simulink model "Seventh_Order_Polynomial_Clean_Test_Harness"  (R2021b)
settings: Solver=FixedStepDiscrete  StartTime=0.0  StopTime=56  FixedStep=0.001  RelTol=1e-3
model workspace (MAT data in the model file):
  mwTaskManagerKernelLatency = 0
libraries: simulink_extras x2
settings Model: Creator=salva  LastModifiedBy=salva
settings DataIOCC: ReturnWorkspaceOutputsName=septic_out
settings OptimizationCC: DefaultParameterBehavior=Inlined  DefaultUnderspecifiedDataType=single  EnhancedBackFolding=on  PassReuseOutputArgsAs=Individual arguments  ZeroExternalMemoryAtStartup=off  ZeroInternalMemoryAtStartup=off  MaxStackSize=64  OptimizeBlockOrder=speed  DifferentSizesBufferReuse=on  OptimizationCustomize=off  EfficientTunableParamExpr=on
settings DebuggingCC: ParameterTunabilityLossMsg=error
settings HardwareCC: ProdBitPerChar=16  ProdBitPerInt=16  ProdBitPerPointer=32  ProdBitPerSizeT=32  ProdBitPerPtrDiffT=32  ProdLargestAtomicInteger=Integer  ProdLargestAtomicFloat=None  ProdWordSize=16  ProdHWDeviceType=Texas Instruments->C2000  HardwareBoardFeatureSet=SoCBlockset
settings ModelReferenceCC: ModelReferenceNumInstancesAllowed=Single
settings SFSimCC: MATLABDynamicMemAlloc=off
settings RTWCC: Description=Embedded Coder  SystemTargetFile=ert.tlc  TemplateMakefile=ert_default_tmf
settings CodeAppCC: ForceParamTrailComments=on  IgnoreCustomStorageClasses=off  OperatorAnnotations=on  SimulinkDataObjDesc=on  SFDataObjDesc=on  InsertBlockDesc=on
settings ERTTargetCC: TargetLangStandard=C99 (ISO)  InlinedParameterPlacement=NonHierarchical  ERTCustomFileTemplate=example_file_process.tlc

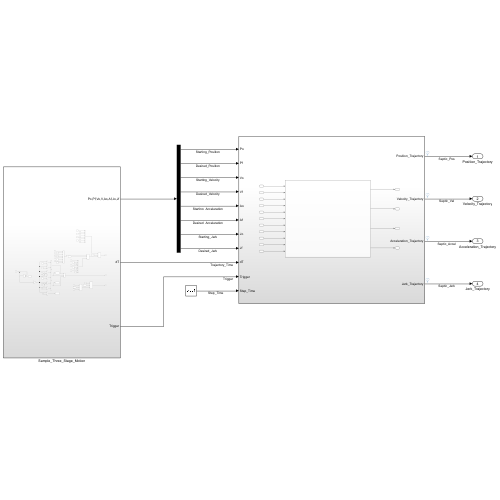
[thumbnail: Simulink's stored preview of the top-level diagram]
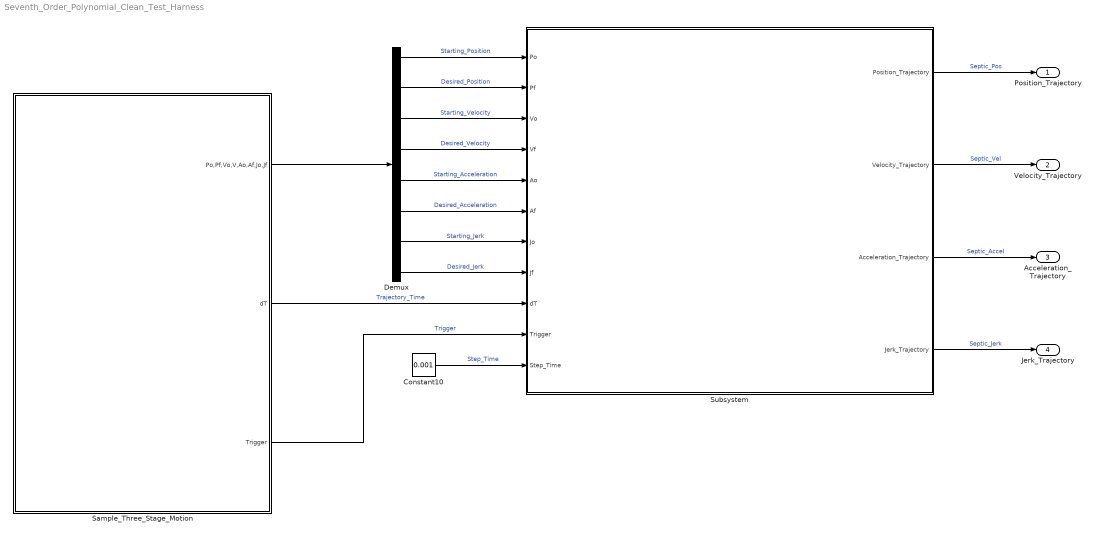
== system Seventh_Order_Polynomial_Clean_Test_Harness ==
  Constant10 : Constant  Value=0.001
  Demux : Demux  Outputs=8
  Sample_Three_Stage_Motion : Subsystem
  Subsystem : Subsystem
  Position_Trajectory : Outport
  Velocity_Trajectory : Outport  Port=2
  Acceleration_Trajectory : Outport  Port=3
  Jerk_Trajectory : Outport  Port=4
  wires:
  Demux/1 -> Subsystem/1(Po)  "Starting_Position"
  Demux/2 -> Subsystem/2(Pf)  "Desired_Position"
  Demux/3 -> Subsystem/3(Vo)  "Starting_Velocity"
  Demux/4 -> Subsystem/4(Vf)  "Desired_Velocity"
  Demux/5 -> Subsystem/5(Ao)  "Starting_Acceleration"
  Demux/6 -> Subsystem/6(Af)  "Desired_Acceleration"
  Demux/7 -> Subsystem/7(Jo)  "Starting_Jerk"
  Demux/8 -> Subsystem/8(Jf)  "Desired_Jerk"
  Constant10/1 -> Subsystem/11(Step_Time)  "Step_Time"
  Subsystem/1(Position_Trajectory) -> Position_Trajectory/1  "Septic_Pos"
  Subsystem/2(Velocity_Trajectory) -> Velocity_Trajectory/1  "Septic_Vel"
  Subsystem/3(Acceleration_Trajectory) -> Acceleration_Trajectory/1  "Septic_Accel"
  Subsystem/4(Jerk_Trajectory) -> Jerk_Trajectory/1  "Septic_Jerk"
  Sample_Three_Stage_Motion/3(Trigger) -> Subsystem/10(Trigger)  "Trigger"
  Sample_Three_Stage_Motion/2(dT) -> Subsystem/9(dT)  "Trajectory_Time"
  Sample_Three_Stage_Motion/1(Po,Pf,Vo,V,Ao,Af,Jo,Jf) -> Demux/1

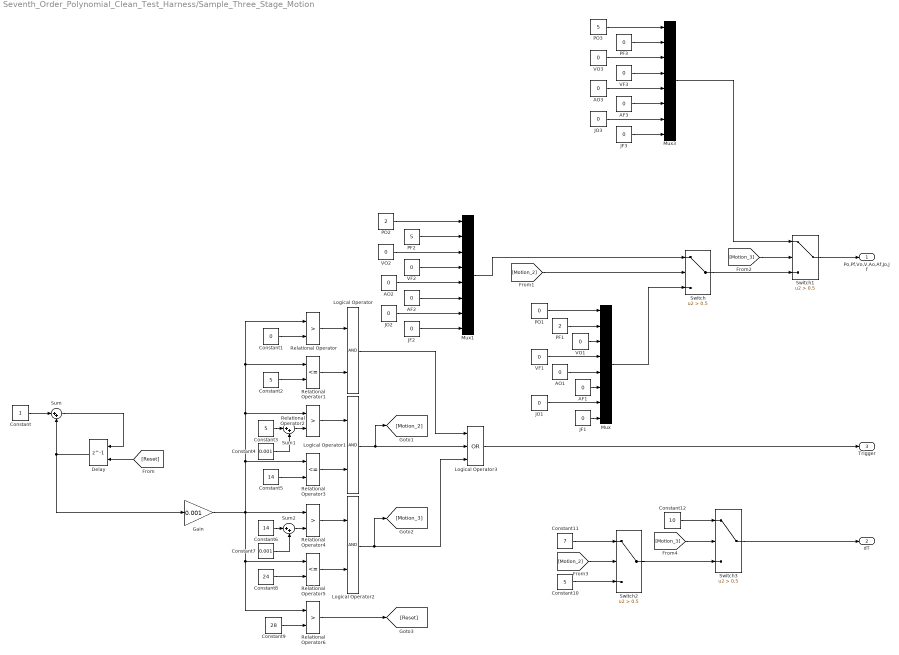
== system Seventh_Order_Polynomial_Clean_Test_Harness/Sample_Three_Stage_Motion ==
  AF1 : Constant  Value=0
  AF2 : Constant  Value=0
  AF3 : Constant  Value=0
  AO1 : Constant  Value=0
  AO2 : Constant  Value=0
  AO3 : Constant  Value=0
  Constant : Constant
  Constant1 : Constant  Value=0
  Constant10 : Constant  Value=5
  Constant11 : Constant  Value=7
  Constant12 : Constant  Value=10
  Constant2 : Constant  Value=5
  Constant3 : Constant  Value=5
  Constant4 : Constant  Value=0.001
  Constant5 : Constant  Value=14
  Constant6 : Constant  Value=14
  Constant7 : Constant  Value=0.001
  Constant8 : Constant  Value=24
  Constant9 : Constant  Value=28
  Delay : Delay  DelayLength=1  ExternalReset=Rising
      settings: InputPortMap=u0,r5
  Gain : Gain  Gain=0.001
  JF1 : Constant  Value=0
  JF2 : Constant  Value=0
  JF3 : Constant  Value=0
  JO1 : Constant  Value=0
  JO2 : Constant  Value=0
  JO3 : Constant  Value=0
  Logical Operator : Logic  AllPortsSameDT=off  OutDataTypeStr=boolean
  Logical Operator1 : Logic  AllPortsSameDT=off  OutDataTypeStr=boolean
  Logical Operator2 : Logic  AllPortsSameDT=off  OutDataTypeStr=boolean
  Logical Operator3 : Logic  Operator=OR  Inputs=3  AllPortsSameDT=off  OutDataTypeStr=boolean
  Mux : Mux  Inputs=8
  Mux1 : Mux  Inputs=8
  Mux3 : Mux  Inputs=8
  PF1 : Constant  Value=2
  PF2 : Constant  Value=5
  PF3 : Constant  Value=0
  PO1 : Constant  Value=0
  PO2 : Constant  Value=2
  PO3 : Constant  Value=5
  Relational Operator{,2,4,6} (4 alike) : RelationalOperator  Operator=>  OutDataTypeStr=boolean  RndMeth=Simplest
  Relational Operator1 : RelationalOperator  Operator=<=  OutDataTypeStr=boolean  RndMeth=Simplest
  Relational Operator3 : RelationalOperator  Operator=<=  OutDataTypeStr=boolean  RndMeth=Simplest
  Relational Operator5 : RelationalOperator  Operator=<=  OutDataTypeStr=boolean  RndMeth=Simplest
  Sum : Sum  Inputs=|++
  Sum1 : Sum  Inputs=|++
  Sum2 : Sum  Inputs=|++
  Switch{,1..3} (4 alike) : Switch  Criteria=u2 > Threshold  Threshold=0.5
  VF1 : Constant  Value=0
  VF2 : Constant  Value=0
  VF3 : Constant  Value=0
  VO1 : Constant  Value=0
  VO2 : Constant  Value=0
  VO3 : Constant  Value=0
  Po,Pf,Vo,V,Ao,Af,Jo,Jf : Outport
  dT : Outport  Port=2
  Trigger : Outport  Port=3
  wires:
  VF2/1 -> Mux1/4
  Delay/1 -> Sum/2, Gain/1
  Sum1/1 -> Relational Operator2/2
  Constant3/1 -> Sum1/1
  Constant1/1 -> Relational Operator/2
  VO2/1 -> Mux1/3
  Gain/1 -> Relational Operator/1, Relational Operator1/1, Relational Operator2/1, Relational Operator3/1, Relational Operator6/1, Relational Operator5/1, Relational Operator4/1
  Switch1/1 -> Po,Pf,Vo,V,Ao,Af,Jo,Jf/1
  Relational Operator3/1 -> Logical Operator1/2
  Switch/1 -> Switch1/3
  Constant/1 -> Sum/1
  Logical Operator2/1 -> [Motion_3], Logical Operator3/3
  Sum2/1 -> Relational Operator4/2
  PO1/1 -> Mux/1
  [Motion_2] -> Switch/2
  VF1/1 -> Mux/4
  Constant6/1 -> Sum2/1
  Constant8/1 -> Relational Operator5/2
  Constant7/1 -> Sum2/2
  Constant9/1 -> Relational Operator6/2
  Relational Operator1/1 -> Logical Operator/2
  PO3/1 -> Mux3/1
  Relational Operator/1 -> Logical Operator/1
  Relational Operator5/1 -> Logical Operator2/2
  [Reset] -> Delay/2
  Mux3/1 -> Switch1/1
  Relational Operator4/1 -> Logical Operator2/1
  Sum/1 -> Delay/1
  Mux1/1 -> Switch/1
  PF3/1 -> Mux3/2
  Constant4/1 -> Sum1/2
  VF3/1 -> Mux3/4
  Logical Operator1/1 -> [Motion_2], Logical Operator3/2
  [Motion_3] -> Switch1/2
  Constant2/1 -> Relational Operator1/2
  VO3/1 -> Mux3/3
  Logical Operator3/1 -> Trigger/1
  Logical Operator/1 -> Logical Operator3/1
  Constant5/1 -> Relational Operator3/2
  Mux/1 -> Switch/3
  PF2/1 -> Mux1/2
  PO2/1 -> Mux1/1
  Relational Operator2/1 -> Logical Operator1/1
  Relational Operator6/1 -> [Reset]
  PF1/1 -> Mux/2
  VO1/1 -> Mux/3
  [Motion_2] -> Switch2/2
  Switch2/1 -> Switch3/3
  [Motion_3] -> Switch3/2
  Constant10/1 -> Switch2/3
  Constant11/1 -> Switch2/1
  Constant12/1 -> Switch3/1
  Switch3/1 -> dT/1
  AO1/1 -> Mux/5
  AF1/1 -> Mux/6
  JO1/1 -> Mux/7
  JF1/1 -> Mux/8
  JO2/1 -> Mux1/7
  JF2/1 -> Mux1/8
  AF2/1 -> Mux1/6
  AO2/1 -> Mux1/5
  JF3/1 -> Mux3/8
  JO3/1 -> Mux3/7
  AO3/1 -> Mux3/5
  AF3/1 -> Mux3/6

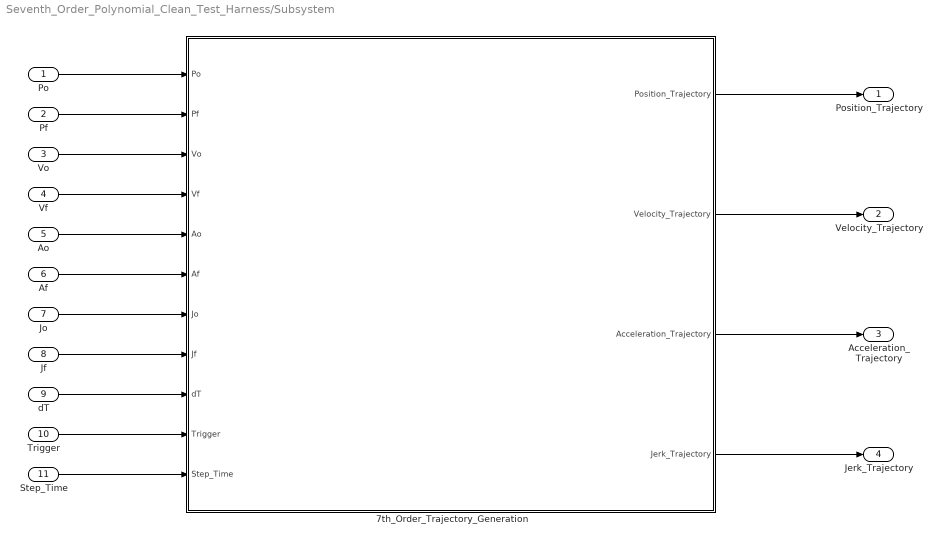
== system Seventh_Order_Polynomial_Clean_Test_Harness/Subsystem ==
  Po : Inport
  Pf : Inport  Port=2
  Vo : Inport  Port=3
  Vf : Inport  Port=4
  Ao : Inport  Port=5
  Af : Inport  Port=6
  Jo : Inport  Port=7
  Jf : Inport  Port=8
  dT : Inport  Port=9
  Trigger : Inport  Port=10
  Step_Time : Inport  Port=11
  7th_Order_Trajectory_Generation : Subsystem
  Position_Trajectory : Outport
  Velocity_Trajectory : Outport  Port=2
  Acceleration_Trajectory : Outport  Port=3
  Jerk_Trajectory : Outport  Port=4
  wires:
  7th_Order_Trajectory_Generation/4(Jerk_Trajectory) -> Jerk_Trajectory/1
  Trigger/1 -> 7th_Order_Trajectory_Generation/10(Trigger)
  Ao/1 -> 7th_Order_Trajectory_Generation/5(Ao)
  Pf/1 -> 7th_Order_Trajectory_Generation/2(Pf)
  Af/1 -> 7th_Order_Trajectory_Generation/6(Af)
  Vo/1 -> 7th_Order_Trajectory_Generation/3(Vo)
  7th_Order_Trajectory_Generation/1(Position_Trajectory) -> Position_Trajectory/1
  dT/1 -> 7th_Order_Trajectory_Generation/9(dT)
  Po/1 -> 7th_Order_Trajectory_Generation/1(Po)
  7th_Order_Trajectory_Generation/2(Velocity_Trajectory) -> Velocity_Trajectory/1
  Vf/1 -> 7th_Order_Trajectory_Generation/4(Vf)
  7th_Order_Trajectory_Generation/3(Acceleration_Trajectory) -> Acceleration_Trajectory/1
  Step_Time/1 -> 7th_Order_Trajectory_Generation/11(Step_Time)
  Jf/1 -> 7th_Order_Trajectory_Generation/8(Jf)
  Jo/1 -> 7th_Order_Trajectory_Generation/7(Jo)

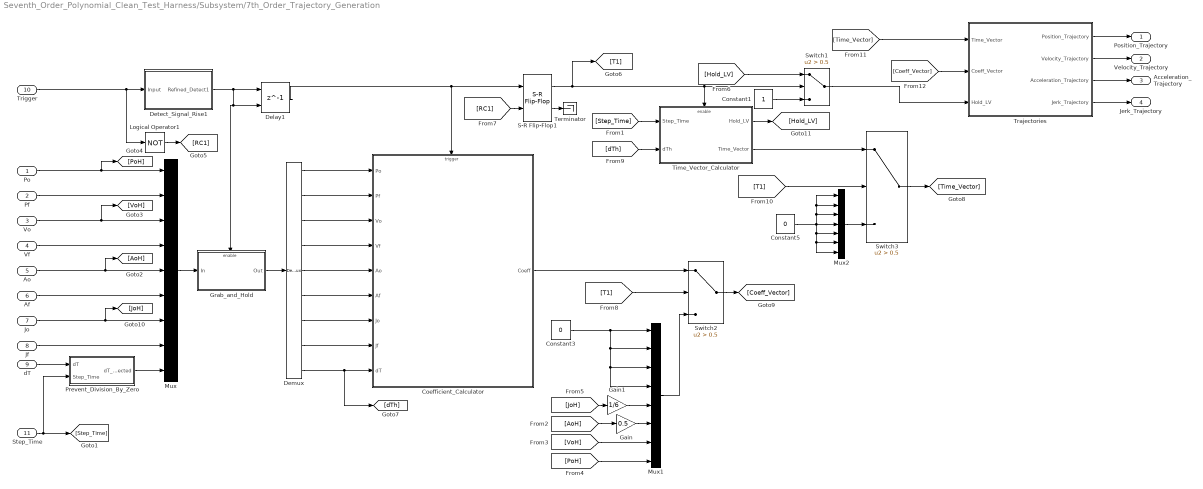
== system Seventh_Order_Polynomial_Clean_Test_Harness/Subsystem/7th_Order_Trajectory_Generation ==
  Po : Inport
  Pf : Inport  Port=2
  Vo : Inport  Port=3
  Vf : Inport  Port=4
  Ao : Inport  Port=5
  Af : Inport  Port=6
  Jo : Inport  Port=7
  Jf : Inport  Port=8
  dT : Inport  Port=9
  Trigger : Inport  Port=10
  Step_Time : Inport  Port=11
  Coefficient_Calculator : Subsystem
  Constant1 : Constant
  Constant3 : Constant  Value=0
  Constant5 : Constant  Value=0
  Delay1 : Delay  DelayLength=1  InitialConditionSource=Input port
      settings: InputPortMap=u0,p4
  Demux : Demux  Outputs=9
  Detect_Signal_Rise1 : Subsystem
  Gain : Gain  Gain=0.5
  Gain1 : Gain  Gain=1/6
  Grab_and_Hold : Subsystem
  Logical Operator1 : Logic  Operator=NOT  AllPortsSameDT=off  OutDataTypeStr=boolean
  Mux : Mux  Inputs=9
  Mux1 : Mux  Inputs=8
  Mux2 : Mux  Inputs=7
  Prevent_Division_By_Zero : Subsystem
  S-R Flip-Flop1 : simulink_extras/Flip Flops/S-R Flip-Flop  initial_condition=0
  Switch1 : Switch  Criteria=u2 > Threshold  Threshold=0.5
  Switch2 : Switch  Criteria=u2 > Threshold  Threshold=0.5
  Switch3 : Switch  Criteria=u2 > Threshold  Threshold=0.5
  Terminator : Terminator
  Time_Vector_Calculator : Subsystem
  Trajectories : Subsystem
  Position_Trajectory : Outport
  Velocity_Trajectory : Outport  Port=2
  Acceleration_Trajectory : Outport  Port=3
  Jerk_Trajectory : Outport  Port=4
  wires:
  Trajectories/2(Velocity_Trajectory) -> Velocity_Trajectory/1
  Trajectories/1(Position_Trajectory) -> Position_Trajectory/1
  [Coeff_Vector] -> Trajectories/2(Coeff_Vector)
  [Time_Vector] -> Trajectories/1(Time_Vector)
  Switch2/1 -> [Coeff_Vector]
  Switch3/1 -> [Time_Vector]
  Constant5/1 -> Mux2/1, Mux2/2, Mux2/3, Mux2/4, Mux2/7, Mux2/6, Mux2/5
  Mux2/1 -> Switch3/3
  Time_Vector_Calculator/2(Time_Vector) -> Switch3/1
  [T1] -> Switch3/2
  [dTh] -> Time_Vector_Calculator/2(dTh)
  [Step_Time] -> Time_Vector_Calculator/1(Step_Time)
  Coefficient_Calculator/1(Coeff) -> Switch2/1
  [T1] -> Switch2/2
  Mux1/1 -> Switch2/3
  S-R Flip-Flop1/1 -> Switch1/2, Time_Vector_Calculator/Enable, [T1]
  S-R Flip-Flop1/2 -> Terminator/1
  [RC1] -> S-R Flip-Flop1/2
  Logical Operator1/1 -> [RC1]
  Delay1/1 -> Coefficient_Calculator/Trigger, S-R Flip-Flop1/1
  Mux/1 -> Grab_and_Hold/1(In)
  Detect_Signal_Rise1/1(Refined_Detect1) -> Delay1/1, Delay1/2, Grab_and_Hold/Enable
  Trigger/1 -> Detect_Signal_Rise1/1(Input), Logical Operator1/1
  Po/1 -> [PoH], Mux/1
  Pf/1 -> Mux/2
  Vo/1 -> [VoH], Mux/3
  Vf/1 -> Mux/4
  Ao/1 -> [AoH], Mux/5
  Af/1 -> Mux/6
  dT/1 -> Prevent_Division_By_Zero/1(dT)
  Grab_and_Hold/1(Out) -> Demux/1
  Trajectories/3(Acceleration_Trajectory) -> Acceleration_Trajectory/1
  Step_Time/1 -> Prevent_Division_By_Zero/2(Step_Time), [Step_Time]
  Prevent_Division_By_Zero/1(dT_Protected) -> Mux/9
  Constant3/1 -> Mux1/4, Mux1/3, Mux1/2, Mux1/1
  [AoH] -> Gain/1
  Jo/1 -> [JoH], Mux/7
  Jf/1 -> Mux/8
  Demux/1 -> Coefficient_Calculator/1(Po)
  Demux/2 -> Coefficient_Calculator/2(Pf)
  Demux/3 -> Coefficient_Calculator/3(Vo)
  Demux/4 -> Coefficient_Calculator/4(Vf)
  Demux/5 -> Coefficient_Calculator/5(Ao)
  Demux/6 -> Coefficient_Calculator/6(Af)
  Demux/7 -> Coefficient_Calculator/7(Jo)
  Demux/8 -> Coefficient_Calculator/8(Jf)
  Demux/9 -> [dTh], Coefficient_Calculator/9(dT)
  [JoH] -> Gain1/1
  Gain1/1 -> Mux1/5
  Gain/1 -> Mux1/6
  [VoH] -> Mux1/7
  [PoH] -> Mux1/8
  Trajectories/4(Jerk_Trajectory) -> Jerk_Trajectory/1
  [Hold_LV] -> Switch1/1
  Switch1/1 -> Trajectories/3(Hold_LV)
  Time_Vector_Calculator/1(Hold_LV) -> [Hold_LV]
  Constant1/1 -> Switch1/3

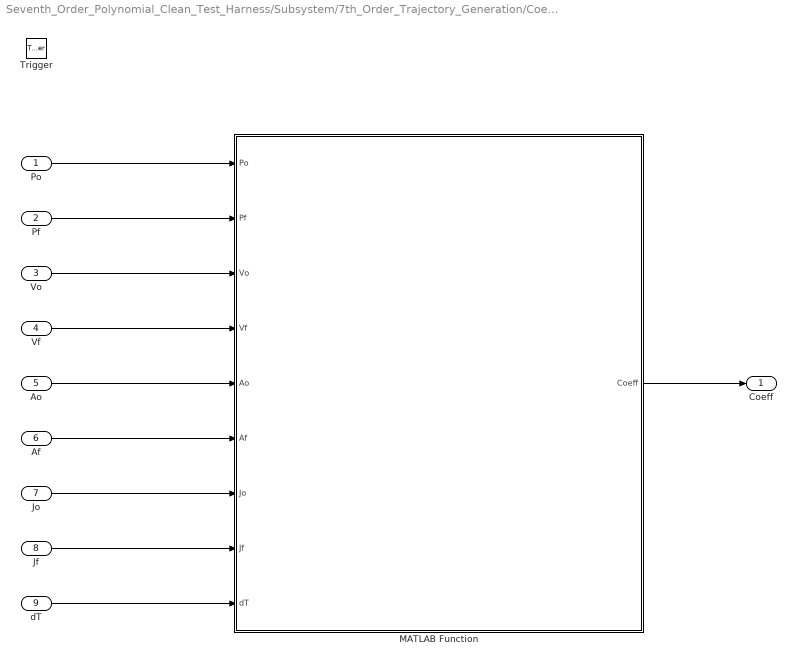
== system Seventh_Order_Polynomial_Clean_Test_Harness/Subsystem/7th_Order_Trajectory_Generation/Coefficient_Calculator ==
  Po : Inport
  Pf : Inport  Port=2
  Vo : Inport  Port=3
  Vf : Inport  Port=4
  Ao : Inport  Port=5
  Af : Inport  Port=6
  Jo : Inport  Port=7
  Jf : Inport  Port=8
  dT : Inport  Port=9
  Trigger : TriggerPort  VariantControl=(inherit)
  MATLAB Function : MATLAB Function  TreatAsAtomicUnit=on
  Coeff : Outport
  wires:
  MATLAB Function/1(Coeff) -> Coeff/1
  Pf/1 -> MATLAB Function/2(Pf)
  Vf/1 -> MATLAB Function/4(Vf)
  Vo/1 -> MATLAB Function/3(Vo)
  Po/1 -> MATLAB Function/1(Po)
  dT/1 -> MATLAB Function/9(dT)
  Ao/1 -> MATLAB Function/5(Ao)
  Af/1 -> MATLAB Function/6(Af)
  Jo/1 -> MATLAB Function/7(Jo)
  Jf/1 -> MATLAB Function/8(Jf)

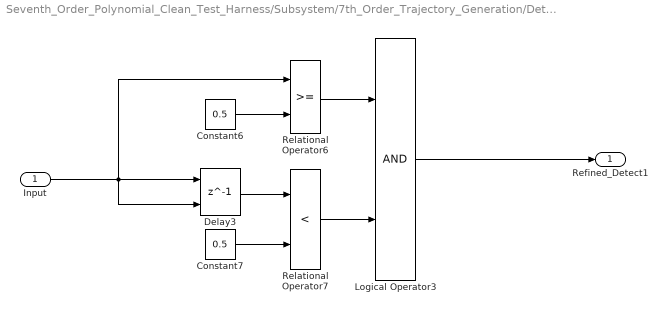
== system Seventh_Order_Polynomial_Clean_Test_Harness/Subsystem/7th_Order_Trajectory_Generation/Detect_Signal_Rise1 ==
  Input : Inport
  Constant6 : Constant  Value=0.5
  Constant7 : Constant  Value=0.5
  Delay3 : Delay  DelayLength=1  InitialConditionSource=Input port
      settings: InputPortMap=u0,p4
  Logical Operator3 : Logic  AllPortsSameDT=off  OutDataTypeStr=boolean
  Relational Operator6 : RelationalOperator  OutDataTypeStr=boolean  RndMeth=Simplest
  Relational Operator7 : RelationalOperator  Operator=<  OutDataTypeStr=boolean  RndMeth=Simplest
  Refined_Detect1 : Outport
  wires:
  Delay3/1 -> Relational Operator7/1
  Relational Operator7/1 -> Logical Operator3/2
  Relational Operator6/1 -> Logical Operator3/1
  Input/1 -> Delay3/2, Delay3/1, Relational Operator6/1
  Constant7/1 -> Relational Operator7/2
  Constant6/1 -> Relational Operator6/2
  Logical Operator3/1 -> Refined_Detect1/1

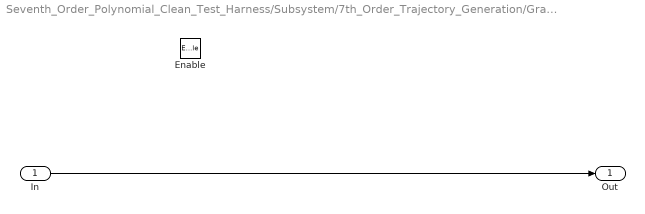
== system Seventh_Order_Polynomial_Clean_Test_Harness/Subsystem/7th_Order_Trajectory_Generation/Grab_and_Hold ==
  In : Inport
  Enable : EnablePort  StatesWhenEnabling=reset
  Out : Outport
  wires:
  In/1 -> Out/1

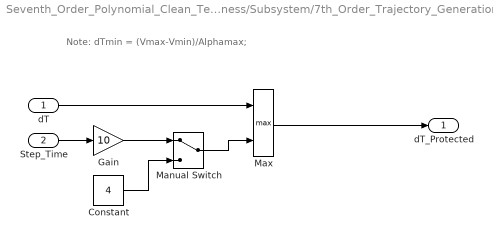
== system Seventh_Order_Polynomial_Clean_Test_Harness/Subsystem/7th_Order_Trajectory_Generation/Prevent_Division_By_Zero ==
  note: Note: dTmin = (Vmax-Vmin)/Alphamax;
  dT : Inport
  Step_Time : Inport  Port=2
  Constant : Constant  Value=4
  Gain : Gain  Gain=10
  Manual Switch : ManualSwitch
  Max : MinMax  Function=max  Inputs=2
  dT_Protected : Outport
  wires:
  dT/1 -> Max/1
  Step_Time/1 -> Gain/1
  Gain/1 -> Manual Switch/1
  Max/1 -> dT_Protected/1
  Manual Switch/1 -> Max/2
  Constant/1 -> Manual Switch/2

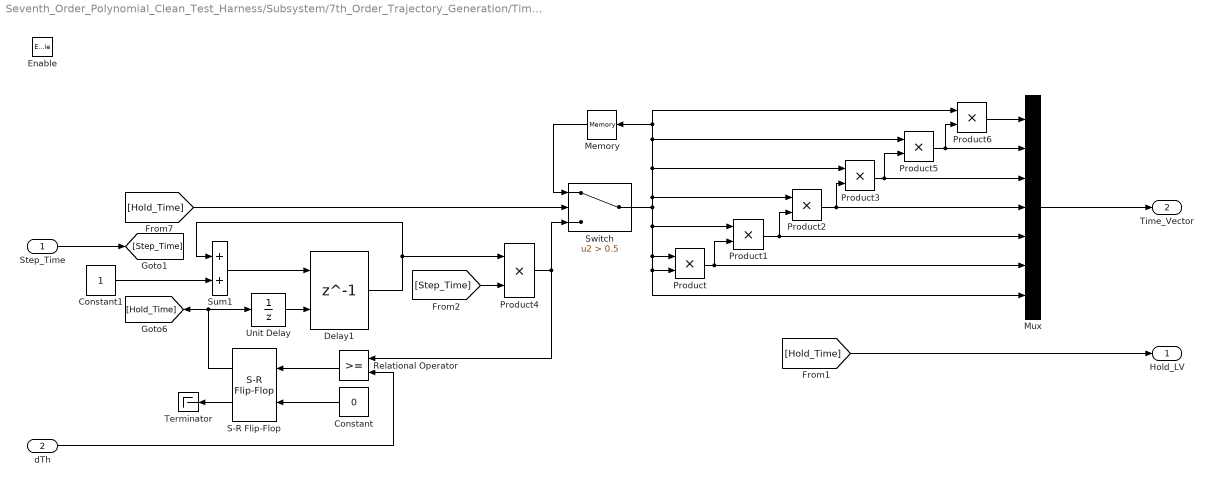
== system Seventh_Order_Polynomial_Clean_Test_Harness/Subsystem/7th_Order_Trajectory_Generation/Time_Vector_Calculator ==
  Step_Time : Inport
  dTh : Inport  Port=2
  Enable : EnablePort  StatesWhenEnabling=reset
  Constant : Constant  Value=0  OutDataTypeStr=boolean
  Constant1 : Constant
  Delay1 : Delay  DelayLength=1  ExternalReset=Level hold
      settings: InputPortMap=u0,r5
  Memory : Memory
  Mux : Mux  Inputs=7
  Product{,1..6} (7 alike) : Product
  Relational Operator : RelationalOperator  OutDataTypeStr=boolean  RndMeth=Simplest
  S-R Flip-Flop : simulink_extras/Flip Flops/S-R Flip-Flop  initial_condition=0
  Sum1 : Sum
  Switch : Switch  Criteria=u2 > Threshold  Threshold=0.5
  Terminator : Terminator
  Unit Delay : UnitDelay  SampleTime=-1  HasFrameUpgradeWarning=on
  Hold_LV : Outport
  Time_Vector : Outport  Port=2
  wires:
  [Hold_Time] -> Hold_LV/1
  Memory/1 -> Switch/1
  Switch/1 -> Product1/1, Product/1, Mux/7, Product/2, Product6/1, Memory/1, Product5/1, Product3/1, Product2/1
  [Hold_Time] -> Switch/2
  Unit Delay/1 -> Delay1/2
  S-R Flip-Flop/1 -> [Hold_Time], Unit Delay/1
  S-R Flip-Flop/2 -> Terminator/1
  Constant/1 -> S-R Flip-Flop/2
  Relational Operator/1 -> S-R Flip-Flop/1
  Mux/1 -> Time_Vector/1
  Product/1 -> Product1/2, Mux/6
  dTh/1 -> Relational Operator/2
  Delay1/1 -> Sum1/1, Product4/1
  Sum1/1 -> Delay1/1
  Product1/1 -> Product2/2, Mux/5
  Product2/1 -> Product3/2, Mux/4
  Step_Time/1 -> [Step_Time]
  Constant1/1 -> Sum1/2
  [Step_Time] -> Product4/2
  Product4/1 -> Switch/3, Relational Operator/1
  Product3/1 -> Product5/2, Mux/3
  Product5/1 -> Product6/2, Mux/2
  Product6/1 -> Mux/1

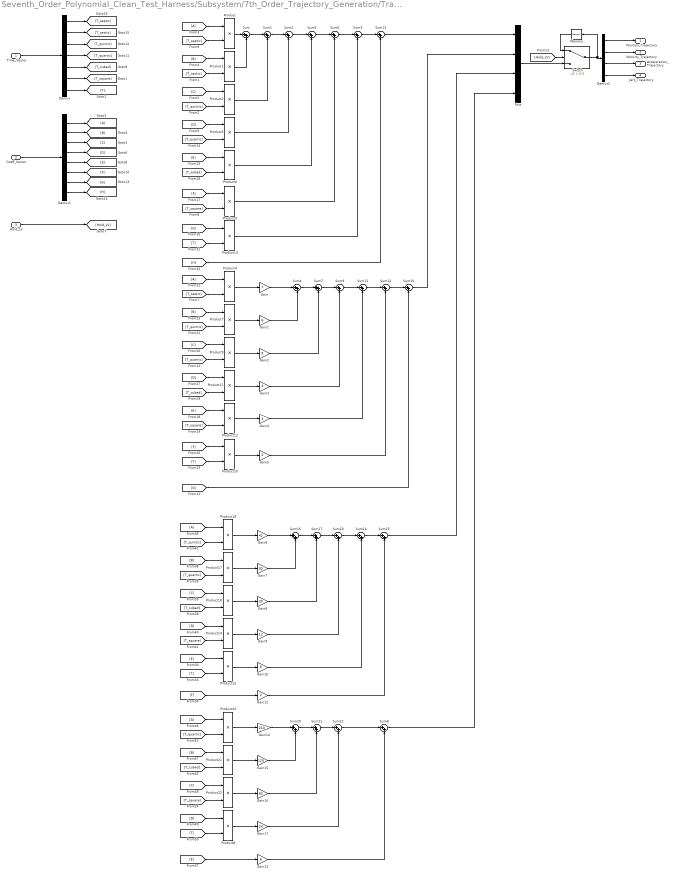
== system Seventh_Order_Polynomial_Clean_Test_Harness/Subsystem/7th_Order_Trajectory_Generation/Trajectories ==
  Time_Vector : Inport
  Coeff_Vector : Inport  Port=2
  Hold_LV : Inport  Port=3
  Demux : Demux  Outputs=7
  Demux1 : Demux  Outputs=8
  Demux2 : Demux
  Gain : Gain  Gain=7
  Gain1 : Gain  Gain=6
  Gain10 : Gain  Gain=6
  Gain11 : Gain  Gain=2
  Gain12 : Gain  Gain=6
  Gain14 : Gain  Gain=210
  Gain15 : Gain  Gain=120
  Gain16 : Gain  Gain=60
  Gain17 : Gain  Gain=24
  Gain2 : Gain  Gain=5
  Gain3 : Gain  Gain=4
  Gain4 : Gain  Gain=3
  Gain5 : Gain  Gain=2
  Gain6 : Gain  Gain=42
  Gain7 : Gain  Gain=30
  Gain8 : Gain  Gain=20
  Gain9 : Gain  Gain=12
  Memory : Memory
  Mux : Mux
  Product{,1..18,20..22} (22 alike) : Product
  Sum{,1..18,20..22} (22 alike) : Sum  Inputs=|++
  Switch : Switch  Criteria=u2 > Threshold  Threshold=0.5
  Position_Trajectory : Outport
  Velocity_Trajectory : Outport  Port=2
  Acceleration_Trajectory : Outport  Port=3
  Jerk_Trajectory : Outport  Port=4
  wires:
  Demux2/2 -> Velocity_Trajectory/1
  Demux2/1 -> Position_Trajectory/1
  [Hold_LV] -> Switch/2
  Memory/1 -> Switch/1
  Switch/1 -> Memory/1, Demux2/1
  Hold_LV/1 -> [Hold_LV]
  Mux/1 -> Switch/3
  Sum1/1 -> Sum2/1
  Product2/1 -> Sum1/2
  [T_quintic] -> Product2/2
  [C] -> Product2/1
  Sum/1 -> Sum1/1
  Product1/1 -> Sum/2
  [T_sextic] -> Product1/2
  [B] -> Product1/1
  Product/1 -> Sum/1
  [T_septic] -> Product/2
  [A] -> Product/1
  Demux1/4 -> [D]
  Demux1/3 -> [C]
  Demux1/2 -> [B]
  Demux1/1 -> [A]
  Coeff_Vector/1 -> Demux1/1
  Time_Vector/1 -> Demux/1
  Demux1/5 -> [E]
  Demux1/6 -> [F]
  [D] -> Product5/1
  [T_quartic] -> Product5/2
  Product5/1 -> Sum2/2
  Sum2/1 -> Sum5/1
  Product6/1 -> Sum5/2
  [E] -> Product6/1
  [T_cubed] -> Product6/2
  Sum5/1 -> Sum6/1
  Demux2/3 -> Acceleration_Trajectory/1
  Demux1/7 -> [G]
  Demux1/8 -> [H]
  Demux/7 -> [T]
  Demux/6 -> [T_square]
  Demux/5 -> [T_cubed]
  Demux/4 -> [T_quartic]
  Demux/3 -> [T_quintic]
  Demux/2 -> [T_sextic]
  Demux/1 -> [T_septic]
  [F] -> Product3/1
  [T_square] -> Product3/2
  Product3/1 -> Sum6/2
  Sum6/1 -> Sum3/1
  [G] -> Product13/1
  [T] -> Product13/2
  Product13/1 -> Sum3/2
  Sum3/1 -> Sum13/1
  [H] -> Sum13/2
  Product10/1 -> Gain5/1
  [T] -> Product10/2
  [F] -> Product10/1
  [G] -> Sum10/2
  Product4/1 -> Gain/1
  [A] -> Product4/1
  Sum4/1 -> Sum7/1
  [E] -> Product12/1
  Product12/1 -> Gain4/1
  Sum11/1 -> Sum12/1
  Sum12/1 -> Sum10/1
  [D] -> Product11/1
  [C] -> Product9/1
  Product11/1 -> Gain3/1
  Sum7/1 -> Sum9/1
  Product9/1 -> Gain2/1
  Product7/1 -> Gain1/1
  Sum9/1 -> Sum11/1
  [B] -> Product7/1
  Gain/1 -> Sum4/1
  [T_sextic] -> Product4/2
  Gain1/1 -> Sum4/2
  [T_quintic] -> Product7/2
  [T_quartic] -> Product9/2
  Gain2/1 -> Sum7/2
  Gain3/1 -> Sum9/2
  [T_cubed] -> Product11/2
  [T_square] -> Product12/2
  Gain4/1 -> Sum11/2
  Gain5/1 -> Sum12/2
  Gain11/1 -> Sum15/2
  Gain10/1 -> Sum14/2
  Sum18/1 -> Sum14/1
  Product14/1 -> Gain9/1
  Product18/1 -> Gain8/1
  [B] -> Product17/1
  Sum17/1 -> Sum18/1
  Sum16/1 -> Sum17/1
  [E] -> Product15/1
  [C] -> Product18/1
  Sum14/1 -> Sum15/1
  Product15/1 -> Gain10/1
  [D] -> Product14/1
  [F] -> Gain11/1
  [T_quintic] -> Product16/2
  [T_cubed] -> Product18/2
  Product17/1 -> Gain7/1
  Gain7/1 -> Sum16/2
  Product16/1 -> Gain6/1
  Gain6/1 -> Sum16/1
  [T_quartic] -> Product17/2
  Gain9/1 -> Sum18/2
  [T_square] -> Product14/2
  Gain8/1 -> Sum17/2
  [T] -> Product15/2
  [A] -> Product16/1
  Sum13/1 -> Mux/1
  Sum10/1 -> Mux/2
  Sum15/1 -> Mux/3
  [A] -> Product20/1
  Gain16/1 -> Sum21/2
  [T] -> Product8/2
  Gain17/1 -> Sum22/2
  [T_cubed] -> Product21/2
  Gain14/1 -> Sum20/1
  Product20/1 -> Gain14/1
  Gain15/1 -> Sum20/2
  Product21/1 -> Gain15/1
  [T_square] -> Product22/2
  [T_quartic] -> Product20/2
  [D] -> Product8/1
  [E] -> Gain12/1
  [C] -> Product22/1
  Sum20/1 -> Sum21/1
  Sum21/1 -> Sum22/1
  [B] -> Product21/1
  Product22/1 -> Gain16/1
  Product8/1 -> Gain17/1
  Sum22/1 -> Sum8/1
  Gain12/1 -> Sum8/2
  Sum8/1 -> Mux/4
  Demux2/4 -> Jerk_Trajectory/1

== matlab function Seventh_Order_Polynomial_Clean_Test_Harness/Subsystem/7th_Order_Trajectory_Generation/Coefficient_Calculator/MATLAB Function ==
  data: Po input; Coeff output; Pf input; Vo input; Vf input; Ao input; Af input; Jo input; Jf input; dT input
function Coeff = solve_septic(Po, Pf, Vo, Vf, Ao, Af, Jo, Jf, dT)

% Position = (A)*dT^7 + (B)*dT^6 + (C)*dT^5 + (D)*dT^4 + (E)*dT^3 + (F)*dT^2 + (G)*dT+ H;
% Velocity = (7*A)*dT^6 + (6*B)*dT^5 + (5*C)*dT^4 + (4*D)*dT^3 + (3*E)*dT^2 + (2*F)*dT+ (G);
% Acceleration = (42*A)*dT^5 + (30*B)*dT^4 + (20*C)*dT^3 + (12*D)*dT^2 + (6*E)*dT + (2*F);
% Jerk = (210*A)*dT^4 + (120*B)*dT^3 + (60*C)*dT^2 + (24*D)*dT + (6*E);
% Where P(t=0) = Po; P(t=dT) = Pf; V(t=0)=Vo; V(t=dT) = Vf; A(t=0) = Ao;
% A(t=dT) = Af; J(t=0) = Jo; J(t=dT) = Jf;

% Calculate 1/dT multiplication to reduce math loading
invdT1 = 1/dT; % 1/dT
invdT2 = invdT1*invdT1; % 1/dT^2
invdT3 = invdT2*invdT1; % 1/dT^3
invdT4 = invdT3*invdT1; % 1/dT^4

% Algebraic Simplications
deltaP = Pf-Po; 
deltaV = Vf-Vo; 
deltaA = Af-Ao;
deltaJ = Jf-Jo;


% Calculate Coefficients
H = Po;
G = Vo;
F = 0.5*Ao;
E = Jo/6;
D = invdT1*(-((5*Jo+deltaJ)/6) + (2.5*(deltaA-Ao)*invdT1) - (5*((7*Vo)+(3*deltaV))*invdT2) + (35*deltaP)*invdT3);
C = invdT2*(((3*Jo+deltaJ)/2) + ((3*Ao-7*deltaA)*invdT1) + (3*((28*Vo)+(13*deltaV))*invdT2) - (84*deltaP)*invdT3);
B = invdT3*((-(7*Jo+3*deltaJ)/6) + (0.5*(13*deltaA-2*Ao)*invdT1) - (2*((35*Vo)+(17*deltaV))*invdT2) + (70*deltaP)*invdT3);
A = invdT4*(((2*Jo+deltaJ)/6) + (-2*deltaA*invdT1) + (10*((2*Vo)+(deltaV))*invdT2) - (20*deltaP)*invdT3);


% Output Coefficients
Coeff = [A,B,C,D,E,F,G,H];
